simulink model "HVDC_VSC_1CPUcore_dcpl"  (Simulink 8.4)
settings: Solver=ode3  SolverMode=SingleTasking  StartTime=0.0  StopTime=70.0  FixedStep=Ts_Power  RelTol=1e-3  AbsTol=1e-2
PreLoadFcn:
  | Ts_Power=50e-6; Ts_Control=1*Ts_Power; init_cosim_IA; startup_transients_hvdc_vsc;
PostLoadFcn:
  | Ts_Power=50e-6; Ts_Control=1*Ts_Power; init_cosim_IA; startup_transients_hvdc_vsc;
InitFcn:
  | Ts_Power=50e-6; Ts_Control=1*Ts_Power; init_cosim_IA; startup_transients_hvdc_vsc;
undefined symbols (not defined in the file): CLARK, D1, Delta, dPref1_2, dPref1_2_rlimit, gcbh, h, intfDelay, level, lib_mesures, magnitude, ResistanceM, rte_drive_private_lib, rte_tsb3level_hiz_rect_cb, sps_rtmsupport, t_deblock_Pref1, t_deblock_Udref2, t_dPref1_2, t_SwitchITMIdc, t_SwitchITMVdc, Ts_intf, TSB3_hiZR
libraries: powerlib x183, spsVIMeasurementModel x102, powerlib_extras x71, powerlib_meascontrol x50, rteventslib x26, op_dpl_lib x20, rtlab x14, sps_avr x6, artemis x1
(part 3 of 13)

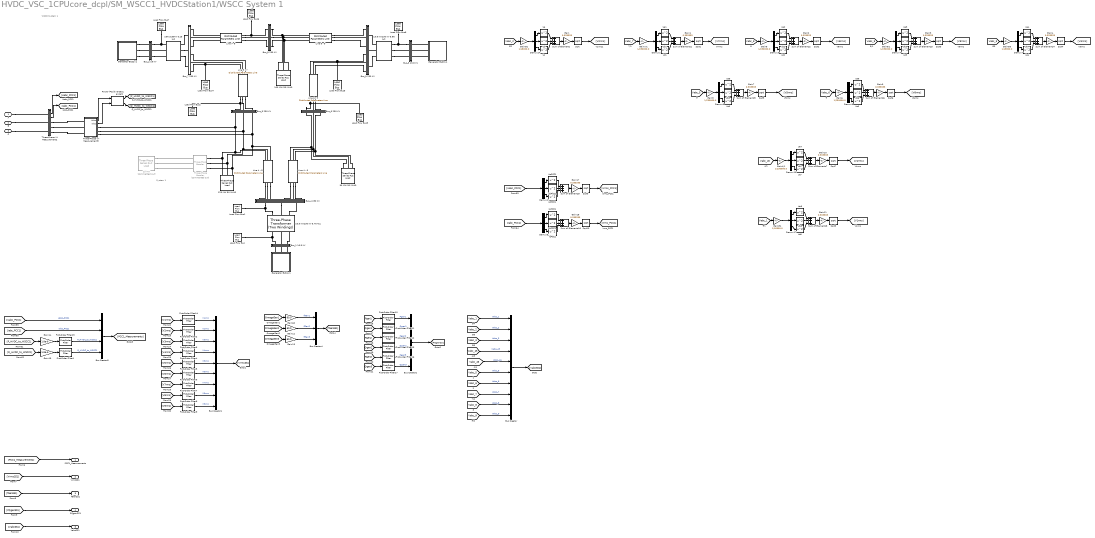
== system HVDC_VSC_1CPUcore_dcpl/SM_WSCC1_HVDCStation1/WSCC System 1 ==
  note: System 1
  note: WSCC System 1
  " Line 4 - 6" : op_dpl_lib/Distributed Parameters Line  SimulationMode=ARTEMIS model  Phases=3  Frequency=60  Resistance=[0.08993 0.224825]  Inductance="[1.41e-3  3.22e-3]"  Capacitance=[7.922e-9 4.74e-9]  Length=100  Measurements=None
  " Line 6 - 9" : op_dpl_lib/Distributed Parameters Line  SimulationMode=ARTEMIS model  Phases=3  Frequency=60  Resistance=[0.20631 0.5157]  Inductance="[2.38e-3  6.09e-3]"  Capacitance=[17.95e-9 10.55e-9]  Length=100  Measurements=None
  100 MW 35 MVAR : powerlib/Elements/Three-Phase Series RLC Load  LConnTagsString=A|B|C  Configuration=Y (grounded)  NominalVoltage=(230000)*1.01601  NominalFrequency=60  ActivePower=100e6  InductivePower=35e6  CapacitivePower=0  Measurements=None  LoadType=constant PQ
  125 MW 50 MVAR : powerlib/Elements/Three-Phase Series RLC Load  LConnTagsString=A|B|C  Configuration=Y (grounded)  NominalVoltage=(230000)*0.996126  NominalFrequency=60  ActivePower=125e6  InductivePower=50e6  CapacitivePower=0  Measurements=None  LoadType=constant PQ
  13.8 KV/230 KV 5.86 %Z : powerlib/Elements/Three-Phase Transformer (Two Windings)  Winding1Connection=Yg  UNITS=pu  NominalPower=[ 128e6 , 60 ]  Winding1=[ 13.8e3 , 1e-6 , 0.0 ]  Winding2Connection=Yg  Winding2=[ 230e3 , 1e-6, 0.075008 ]  SetSaturation=off  Rm=inf  Lm=inf  Saturation=[ 0,0 ; 0.0024,1.2 ; 1.0,1.52 ]  Hysteresis=off  DataFile='hysteresis'  SetInitialFlux=off  InitialFluxes=[ 0.8 , -0.8 , 0.7 ]  Measurements=None  MoreParameters=off  BreakLoop=off  DataType=off  TransfoNumber=1
  "16.5 KV/230 KV 5.76 %Z     " : powerlib/Elements/Three-Phase Transformer (Two Windings)  Winding1Connection=Yg  UNITS=pu  NominalPower=[ 247.5e6 , 60 ]  Winding1=[ 16.5e3 , 1e-6, 0.0 ]  Winding2Connection=Yg  Winding2=[ 230e3 ,1e-6, 0.14256 ]  SetSaturation=off  Rm=inf  Lm=inf  Saturation=[ 0,0 ; 0.0024,1.2 ; 1.0,1.52 ]  Hysteresis=off  DataFile='hysteresis'  SetInitialFlux=off  InitialFluxes=[ 0.8 , -0.8 , 0.7 ]  Measurements=None  MoreParameters=off  BreakLoop=off  DataType=off  TransfoNumber=1
  18KV/230KV 6.25 %Z : powerlib/Elements/Three-Phase Transformer (Two Windings)  Winding1Connection=Yg  UNITS=pu  NominalPower=[ 192e6 , 60 ]  Winding1=[ 18e3 , 1e-6 , 0.0 ]  Winding2Connection=Yg  Winding2=[ 230e3 , 1e-6, 0.12 ]  SetSaturation=off  Rm=inf  Lm=inf  Saturation=[ 0,0 ; 0.0024,1.2 ; 1.0,1.52 ]  Hysteresis=off  DataFile='hysteresis'  SetInitialFlux=off  InitialFluxes=[ 0.8 , -0.8 , 0.7 ]  Measurements=None  MoreParameters=off  BreakLoop=off  DataType=off  TransfoNumber=1
  25 MW : powerlib/Elements/Three-Phase Series RLC Load  Commented=on  LConnTagsString=A|B|C  Configuration=Y (grounded)  NominalVoltage=230000  NominalFrequency=60  ActivePower=25e6  InductivePower=0  CapacitivePower=0  Measurements=None  LoadType=constant PQ
  90 MW 30 MVAR : powerlib/Elements/Three-Phase Series RLC Load  LConnTagsString=A|B|C  Configuration=Y (grounded)  NominalVoltage=(230000)*1.01311  NominalFrequency=60  ActivePower=90e6  InductivePower=30e6  CapacitivePower=0  Measurements=None  LoadType=constant PQ
  Bus Creator : BusCreator  Inputs=10
  Bus Creator1 : BusCreator  Inputs=9
  Bus Creator2 : BusCreator  Inputs=6
  Bus Creator4 : BusCreator  Inputs=3
  Bus Creator5 : BusCreator
  Bus_1 16.5 KV : Subsystem  DialogController=POWERSYS.PowerSysDialog  LoadFcn=sps_rtmsupport('LoadFcn',gcbh);  StartFcn=sps_rtmsupport('StartFcn',gcbh);  StopFcn=sps_rtmsupport('StopFcn',gcbh);  mask(Three-Phase VI Measurement){VoltageMeasurement=phase-to-phase, SetLabelV=on, LabelV=Vabc_1, Vpu=off, VpuLL=off, CurrentMeasurement=yes, SetLabelI=on, LabelI=Iabc_1, Ipu=off, Pbase=100e6, Vbase=16.5e3, OutputType=Complex, PhasorSimulation=off, PSBequivalent=0}
      mask prompts: VoltageMeasurement "Voltage measurement"; SetLabelV "Use a label"; LabelV "Signal label  (use a From block to collect this signal)"; Vpu "Voltages in pu,  based on peak value of nominal phase-to-ground voltage"; VpuLL "Voltages in pu,  based on peak value of nominal phase-to-phase  voltage"; CurrentMeasurement "Current measurement"; SetLabelI "Use a label"; LabelI "Signal label  (use a From block to collect this signal)"; Ipu "Currents in pu"; Pbase "Base power ( VA 3 phase)"; Vbase "Nominal voltage used for pu measurement (Vrms phase-phase) :"; OutputType "Output signals in:"; PhasorSimulation "Phasor simulation (internal use)"; PSBequivalent "Equivalent circuit (internal use)"
      mask help:
      | Ideal three-phase voltage and current measurements.
      |
      | The block can output the voltages and currents in per unit values or in volts and amperes.
      mask init: same as HVDC_VSC_1CPUcore_dcpl/SM_WSCC1_HVDCStation1/B1
      settings: CopyFcn=sps_rtmsupport('CopyFcn',gcbh); powericon('ThreePhaseVIMeasurementCopy',gcb)  DeleteFcn=sps_rtmsupport('DeleteFcn',gcbh);  UndoDeleteFcn=sps_rtmsupport('UndoDeleteFcn',gcbh);  ModelCloseFcn=sps_rtmsupport('ModelCloseFcn',gcbh);  PreSaveFcn="sps_rtmsupport('PreSaveFcn',gcbh);  set_param(gcb,'LinkStatus','restore')"  PostSaveFcn=sps_rtmsupport('PostSaveFcn',gcbh);  NameChangeFcn=sps_rtmsupport('NameChangeFcn',gcbh);  PreCopyFcn=sps_rtmsupport('PreCopyFcn',gcbh);  OpenFcn=sps_rtmsupport('OpenFcn',gcbh, [1 2 4 5 6 7 9 -12 13]);  CloseFcn=sps_rtmsupport('CloseFcn',gcbh);  PreDeleteFcn=sps_rtmsupport('PreDeleteFcn',gcbh);
      mask Help: helpview(psbhelp)
      mask TypeOptions VoltageMeasurement: no | phase-to-ground | phase-to-phase
      mask Callback VoltageMeasurement: powericon('ThreePhaseVIMeasurementCback',gcb,'Vselector');
      mask Callback SetLabelV: powericon('ThreePhaseVIMeasurementCback',gcb,'');
      mask Callback Vpu: powericon('ThreePhaseVIMeasurementCback',gcb,'Vpu');
      mask Callback VpuLL: powericon('ThreePhaseVIMeasurementCback',gcb,'VpuLL');
      mask TypeOptions CurrentMeasurement: no | yes
      mask Callback CurrentMeasurement: powericon('ThreePhaseVIMeasurementCback',gcb,'');
      mask Callback SetLabelI: powericon('ThreePhaseVIMeasurementCback',gcb,'');
      mask Callback LabelI: powericon('ThreePhaseVIMeasurementCback',gcb,'');
      mask Callback Ipu: powericon('ThreePhaseVIMeasurementCback',gcb,'');
      mask TypeOptions OutputType: Complex | Real-Imag | Magnitude-Angle | Magnitude
  Bus_2 18 KV : Subsystem  DialogController=POWERSYS.PowerSysDialog  LoadFcn=sps_rtmsupport('LoadFcn',gcbh);  StartFcn=sps_rtmsupport('StartFcn',gcbh);  StopFcn=sps_rtmsupport('StopFcn',gcbh);  mask(Three-Phase VI Measurement){VoltageMeasurement=phase-to-phase, SetLabelV=on, LabelV=Vabc_2, Vpu=off, VpuLL=off, CurrentMeasurement=yes, SetLabelI=on, LabelI=Iabc_2, Ipu=off, Pbase=100e6, Vbase=18e3, OutputType=Complex, PhasorSimulation=off, PSBequivalent=0}
      mask prompts: VoltageMeasurement "Voltage measurement"; SetLabelV "Use a label"; LabelV "Signal label  (use a From block to collect this signal)"; Vpu "Voltages in pu,  based on peak value of nominal phase-to-ground voltage"; VpuLL "Voltages in pu,  based on peak value of nominal phase-to-phase  voltage"; CurrentMeasurement "Current measurement"; SetLabelI "Use a label"; LabelI "Signal label  (use a From block to collect this signal)"; Ipu "Currents in pu"; Pbase "Base power ( VA 3 phase)"; Vbase "Nominal voltage used for pu measurement (Vrms phase-phase) :"; OutputType "Output signals in:"; PhasorSimulation "Phasor simulation (internal use)"; PSBequivalent "Equivalent circuit (internal use)"
      mask help:
      | Ideal three-phase voltage and current measurements.
      |
      | The block can output the voltages and currents in per unit values or in volts and amperes.
      mask init: same as HVDC_VSC_1CPUcore_dcpl/SM_WSCC1_HVDCStation1/B1
      settings: CopyFcn=sps_rtmsupport('CopyFcn',gcbh); powericon('ThreePhaseVIMeasurementCopy',gcb)  DeleteFcn=sps_rtmsupport('DeleteFcn',gcbh);  UndoDeleteFcn=sps_rtmsupport('UndoDeleteFcn',gcbh);  ModelCloseFcn=sps_rtmsupport('ModelCloseFcn',gcbh);  PreSaveFcn="sps_rtmsupport('PreSaveFcn',gcbh);  set_param(gcb,'LinkStatus','restore')"  PostSaveFcn=sps_rtmsupport('PostSaveFcn',gcbh);  NameChangeFcn=sps_rtmsupport('NameChangeFcn',gcbh);  PreCopyFcn=sps_rtmsupport('PreCopyFcn',gcbh);  OpenFcn=sps_rtmsupport('OpenFcn',gcbh, [1 2 4 5 6 7 9 -12 13]);  CloseFcn=sps_rtmsupport('CloseFcn',gcbh);  PreDeleteFcn=sps_rtmsupport('PreDeleteFcn',gcbh);
      mask Help: helpview(psbhelp)
      mask TypeOptions VoltageMeasurement: no | phase-to-ground | phase-to-phase
      mask Callback VoltageMeasurement: powericon('ThreePhaseVIMeasurementCback',gcb,'Vselector');
      mask Callback SetLabelV: powericon('ThreePhaseVIMeasurementCback',gcb,'');
      mask Callback Vpu: powericon('ThreePhaseVIMeasurementCback',gcb,'Vpu');
      mask Callback VpuLL: powericon('ThreePhaseVIMeasurementCback',gcb,'VpuLL');
      mask TypeOptions CurrentMeasurement: no | yes
      mask Callback CurrentMeasurement: powericon('ThreePhaseVIMeasurementCback',gcb,'');
      mask Callback SetLabelI: powericon('ThreePhaseVIMeasurementCback',gcb,'');
      mask Callback LabelI: powericon('ThreePhaseVIMeasurementCback',gcb,'');
      mask Callback Ipu: powericon('ThreePhaseVIMeasurementCback',gcb,'');
      mask TypeOptions OutputType: Complex | Real-Imag | Magnitude-Angle | Magnitude
  Bus_3 13.8 KV : Subsystem  DialogController=POWERSYS.PowerSysDialog  LoadFcn=sps_rtmsupport('LoadFcn',gcbh);  StartFcn=sps_rtmsupport('StartFcn',gcbh);  StopFcn=sps_rtmsupport('StopFcn',gcbh);  mask(Three-Phase VI Measurement){VoltageMeasurement=phase-to-phase, SetLabelV=on, LabelV=Vabc_3, Vpu=off, VpuLL=off, CurrentMeasurement=yes, SetLabelI=on, LabelI=Iabc_3, Ipu=off, Pbase=100e6, Vbase=13.8e3, OutputType=Complex, PhasorSimulation=off, PSBequivalent=0}
      mask prompts: VoltageMeasurement "Voltage measurement"; SetLabelV "Use a label"; LabelV "Signal label  (use a From block to collect this signal)"; Vpu "Voltages in pu,  based on peak value of nominal phase-to-ground voltage"; VpuLL "Voltages in pu,  based on peak value of nominal phase-to-phase  voltage"; CurrentMeasurement "Current measurement"; SetLabelI "Use a label"; LabelI "Signal label  (use a From block to collect this signal)"; Ipu "Currents in pu"; Pbase "Base power ( VA 3 phase)"; Vbase "Nominal voltage used for pu measurement (Vrms phase-phase) :"; OutputType "Output signals in:"; PhasorSimulation "Phasor simulation (internal use)"; PSBequivalent "Equivalent circuit (internal use)"
      mask help:
      | Ideal three-phase voltage and current measurements.
      |
      | The block can output the voltages and currents in per unit values or in volts and amperes.
      mask init: same as HVDC_VSC_1CPUcore_dcpl/SM_WSCC1_HVDCStation1/B1
      settings: CopyFcn=sps_rtmsupport('CopyFcn',gcbh); powericon('ThreePhaseVIMeasurementCopy',gcb)  DeleteFcn=sps_rtmsupport('DeleteFcn',gcbh);  UndoDeleteFcn=sps_rtmsupport('UndoDeleteFcn',gcbh);  ModelCloseFcn=sps_rtmsupport('ModelCloseFcn',gcbh);  PreSaveFcn="sps_rtmsupport('PreSaveFcn',gcbh);  set_param(gcb,'LinkStatus','restore')"  PostSaveFcn=sps_rtmsupport('PostSaveFcn',gcbh);  NameChangeFcn=sps_rtmsupport('NameChangeFcn',gcbh);  PreCopyFcn=sps_rtmsupport('PreCopyFcn',gcbh);  OpenFcn=sps_rtmsupport('OpenFcn',gcbh, [1 2 4 5 6 7 9 -12 13]);  CloseFcn=sps_rtmsupport('CloseFcn',gcbh);  PreDeleteFcn=sps_rtmsupport('PreDeleteFcn',gcbh);
      mask Help: helpview(psbhelp)
      mask TypeOptions VoltageMeasurement: no | phase-to-ground | phase-to-phase
      mask Callback VoltageMeasurement: powericon('ThreePhaseVIMeasurementCback',gcb,'Vselector');
      mask Callback SetLabelV: powericon('ThreePhaseVIMeasurementCback',gcb,'');
      mask Callback Vpu: powericon('ThreePhaseVIMeasurementCback',gcb,'Vpu');
      mask Callback VpuLL: powericon('ThreePhaseVIMeasurementCback',gcb,'VpuLL');
      mask TypeOptions CurrentMeasurement: no | yes
      mask Callback CurrentMeasurement: powericon('ThreePhaseVIMeasurementCback',gcb,'');
      mask Callback SetLabelI: powericon('ThreePhaseVIMeasurementCback',gcb,'');
      mask Callback LabelI: powericon('ThreePhaseVIMeasurementCback',gcb,'');
      mask Callback Ipu: powericon('ThreePhaseVIMeasurementCback',gcb,'');
      mask TypeOptions OutputType: Complex | Real-Imag | Magnitude-Angle | Magnitude
  Bus_4 230 KV : Subsystem
  Bus_5 230 KV : Subsystem  DialogController=POWERSYS.PowerSysDialog  LoadFcn=sps_rtmsupport('LoadFcn',gcbh);  StartFcn=sps_rtmsupport('StartFcn',gcbh);  StopFcn=sps_rtmsupport('StopFcn',gcbh);  mask(Three-Phase VI Measurement){VoltageMeasurement=phase-to-phase, SetLabelV=on, LabelV=Vabc_5, Vpu=off, VpuLL=off, CurrentMeasurement=yes, SetLabelI=on, LabelI=Iabc_5, Ipu=off, Pbase=100e6, Vbase=230e3, OutputType=Complex, PhasorSimulation=off, PSBequivalent=0}
      mask prompts: VoltageMeasurement "Voltage measurement"; SetLabelV "Use a label"; LabelV "Signal label  (use a From block to collect this signal)"; Vpu "Voltages in pu,  based on peak value of nominal phase-to-ground voltage"; VpuLL "Voltages in pu,  based on peak value of nominal phase-to-phase  voltage"; CurrentMeasurement "Current measurement"; SetLabelI "Use a label"; LabelI "Signal label  (use a From block to collect this signal)"; Ipu "Currents in pu"; Pbase "Base power ( VA 3 phase)"; Vbase "Nominal voltage used for pu measurement (Vrms phase-phase) :"; OutputType "Output signals in:"; PhasorSimulation "Phasor simulation (internal use)"; PSBequivalent "Equivalent circuit (internal use)"
      mask help:
      | Ideal three-phase voltage and current measurements.
      |
      | The block can output the voltages and currents in per unit values or in volts and amperes.
      mask init: same as HVDC_VSC_1CPUcore_dcpl/SM_WSCC1_HVDCStation1/B1
      settings: CopyFcn=sps_rtmsupport('CopyFcn',gcbh); powericon('ThreePhaseVIMeasurementCopy',gcb)  DeleteFcn=sps_rtmsupport('DeleteFcn',gcbh);  UndoDeleteFcn=sps_rtmsupport('UndoDeleteFcn',gcbh);  ModelCloseFcn=sps_rtmsupport('ModelCloseFcn',gcbh);  PreSaveFcn="sps_rtmsupport('PreSaveFcn',gcbh);  set_param(gcb,'LinkStatus','restore')"  PostSaveFcn=sps_rtmsupport('PostSaveFcn',gcbh);  NameChangeFcn=sps_rtmsupport('NameChangeFcn',gcbh);  PreCopyFcn=sps_rtmsupport('PreCopyFcn',gcbh);  OpenFcn=sps_rtmsupport('OpenFcn',gcbh, [1 2 4 5 6 7 9 -12 13]);  CloseFcn=sps_rtmsupport('CloseFcn',gcbh);  PreDeleteFcn=sps_rtmsupport('PreDeleteFcn',gcbh);
      mask Help: helpview(psbhelp)
      mask TypeOptions VoltageMeasurement: no | phase-to-ground | phase-to-phase
      mask Callback VoltageMeasurement: powericon('ThreePhaseVIMeasurementCback',gcb,'Vselector');
      mask Callback SetLabelV: powericon('ThreePhaseVIMeasurementCback',gcb,'');
      mask Callback Vpu: powericon('ThreePhaseVIMeasurementCback',gcb,'Vpu');
      mask Callback VpuLL: powericon('ThreePhaseVIMeasurementCback',gcb,'VpuLL');
      mask TypeOptions CurrentMeasurement: no | yes
      mask Callback CurrentMeasurement: powericon('ThreePhaseVIMeasurementCback',gcb,'');
      mask Callback SetLabelI: powericon('ThreePhaseVIMeasurementCback',gcb,'');
      mask Callback LabelI: powericon('ThreePhaseVIMeasurementCback',gcb,'');
      mask Callback Ipu: powericon('ThreePhaseVIMeasurementCback',gcb,'');
      mask TypeOptions OutputType: Complex | Real-Imag | Magnitude-Angle | Magnitude
  Bus_6 230 KV : Subsystem  DialogController=POWERSYS.PowerSysDialog  LoadFcn=sps_rtmsupport('LoadFcn',gcbh);  StartFcn=sps_rtmsupport('StartFcn',gcbh);  StopFcn=sps_rtmsupport('StopFcn',gcbh);  mask(Three-Phase VI Measurement){VoltageMeasurement=phase-to-phase, SetLabelV=on, LabelV=Vabc_6, Vpu=off, VpuLL=off, CurrentMeasurement=yes, SetLabelI=on, LabelI=Iabc_6, Ipu=off, Pbase=100e6, Vbase=230e3, OutputType=Complex, PhasorSimulation=off, PSBequivalent=0}
      mask prompts: VoltageMeasurement "Voltage measurement"; SetLabelV "Use a label"; LabelV "Signal label  (use a From block to collect this signal)"; Vpu "Voltages in pu,  based on peak value of nominal phase-to-ground voltage"; VpuLL "Voltages in pu,  based on peak value of nominal phase-to-phase  voltage"; CurrentMeasurement "Current measurement"; SetLabelI "Use a label"; LabelI "Signal label  (use a From block to collect this signal)"; Ipu "Currents in pu"; Pbase "Base power ( VA 3 phase)"; Vbase "Nominal voltage used for pu measurement (Vrms phase-phase) :"; OutputType "Output signals in:"; PhasorSimulation "Phasor simulation (internal use)"; PSBequivalent "Equivalent circuit (internal use)"
      mask help:
      | Ideal three-phase voltage and current measurements.
      |
      | The block can output the voltages and currents in per unit values or in volts and amperes.
      mask init: same as HVDC_VSC_1CPUcore_dcpl/SM_WSCC1_HVDCStation1/B1
      settings: CopyFcn=sps_rtmsupport('CopyFcn',gcbh); powericon('ThreePhaseVIMeasurementCopy',gcb)  DeleteFcn=sps_rtmsupport('DeleteFcn',gcbh);  UndoDeleteFcn=sps_rtmsupport('UndoDeleteFcn',gcbh);  ModelCloseFcn=sps_rtmsupport('ModelCloseFcn',gcbh);  PreSaveFcn="sps_rtmsupport('PreSaveFcn',gcbh);  set_param(gcb,'LinkStatus','restore')"  PostSaveFcn=sps_rtmsupport('PostSaveFcn',gcbh);  NameChangeFcn=sps_rtmsupport('NameChangeFcn',gcbh);  PreCopyFcn=sps_rtmsupport('PreCopyFcn',gcbh);  OpenFcn=sps_rtmsupport('OpenFcn',gcbh, [1 2 4 5 6 7 9 -12 13]);  CloseFcn=sps_rtmsupport('CloseFcn',gcbh);  PreDeleteFcn=sps_rtmsupport('PreDeleteFcn',gcbh);
      mask Help: helpview(psbhelp)
      mask TypeOptions VoltageMeasurement: no | phase-to-ground | phase-to-phase
      mask Callback VoltageMeasurement: powericon('ThreePhaseVIMeasurementCback',gcb,'Vselector');
      mask Callback SetLabelV: powericon('ThreePhaseVIMeasurementCback',gcb,'');
      mask Callback Vpu: powericon('ThreePhaseVIMeasurementCback',gcb,'Vpu');
      mask Callback VpuLL: powericon('ThreePhaseVIMeasurementCback',gcb,'VpuLL');
      mask TypeOptions CurrentMeasurement: no | yes
      mask Callback CurrentMeasurement: powericon('ThreePhaseVIMeasurementCback',gcb,'');
      mask Callback SetLabelI: powericon('ThreePhaseVIMeasurementCback',gcb,'');
      mask Callback LabelI: powericon('ThreePhaseVIMeasurementCback',gcb,'');
      mask Callback Ipu: powericon('ThreePhaseVIMeasurementCback',gcb,'');
      mask TypeOptions OutputType: Complex | Real-Imag | Magnitude-Angle | Magnitude
  Bus_7 230 KV : Subsystem
  Bus_8 230 KV : Subsystem  DialogController=POWERSYS.PowerSysDialog  LoadFcn=sps_rtmsupport('LoadFcn',gcbh);  StartFcn=sps_rtmsupport('StartFcn',gcbh);  StopFcn=sps_rtmsupport('StopFcn',gcbh);  mask(Three-Phase VI Measurement){VoltageMeasurement=phase-to-phase, SetLabelV=on, LabelV=Vabc_8, Vpu=off, VpuLL=off, CurrentMeasurement=yes, SetLabelI=on, LabelI=Iabc_8, Ipu=off, Pbase=100e6, Vbase=230e3, OutputType=Complex, PhasorSimulation=off, PSBequivalent=0}
      mask prompts: VoltageMeasurement "Voltage measurement"; SetLabelV "Use a label"; LabelV "Signal label  (use a From block to collect this signal)"; Vpu "Voltages in pu,  based on peak value of nominal phase-to-ground voltage"; VpuLL "Voltages in pu,  based on peak value of nominal phase-to-phase  voltage"; CurrentMeasurement "Current measurement"; SetLabelI "Use a label"; LabelI "Signal label  (use a From block to collect this signal)"; Ipu "Currents in pu"; Pbase "Base power ( VA 3 phase)"; Vbase "Nominal voltage used for pu measurement (Vrms phase-phase) :"; OutputType "Output signals in:"; PhasorSimulation "Phasor simulation (internal use)"; PSBequivalent "Equivalent circuit (internal use)"
      mask help:
      | Ideal three-phase voltage and current measurements.
      |
      | The block can output the voltages and currents in per unit values or in volts and amperes.
      mask init: same as HVDC_VSC_1CPUcore_dcpl/SM_WSCC1_HVDCStation1/B1
      settings: CopyFcn=sps_rtmsupport('CopyFcn',gcbh); powericon('ThreePhaseVIMeasurementCopy',gcb)  DeleteFcn=sps_rtmsupport('DeleteFcn',gcbh);  UndoDeleteFcn=sps_rtmsupport('UndoDeleteFcn',gcbh);  ModelCloseFcn=sps_rtmsupport('ModelCloseFcn',gcbh);  PreSaveFcn="sps_rtmsupport('PreSaveFcn',gcbh);  set_param(gcb,'LinkStatus','restore')"  PostSaveFcn=sps_rtmsupport('PostSaveFcn',gcbh);  NameChangeFcn=sps_rtmsupport('NameChangeFcn',gcbh);  PreCopyFcn=sps_rtmsupport('PreCopyFcn',gcbh);  OpenFcn=sps_rtmsupport('OpenFcn',gcbh, [1 2 4 5 6 7 9 -12 13]);  CloseFcn=sps_rtmsupport('CloseFcn',gcbh);  PreDeleteFcn=sps_rtmsupport('PreDeleteFcn',gcbh);
      mask Help: helpview(psbhelp)
      mask TypeOptions VoltageMeasurement: no | phase-to-ground | phase-to-phase
      mask Callback VoltageMeasurement: powericon('ThreePhaseVIMeasurementCback',gcb,'Vselector');
      mask Callback SetLabelV: powericon('ThreePhaseVIMeasurementCback',gcb,'');
      mask Callback Vpu: powericon('ThreePhaseVIMeasurementCback',gcb,'Vpu');
      mask Callback VpuLL: powericon('ThreePhaseVIMeasurementCback',gcb,'VpuLL');
      mask TypeOptions CurrentMeasurement: no | yes
      mask Callback CurrentMeasurement: powericon('ThreePhaseVIMeasurementCback',gcb,'');
      mask Callback SetLabelI: powericon('ThreePhaseVIMeasurementCback',gcb,'');
      mask Callback LabelI: powericon('ThreePhaseVIMeasurementCback',gcb,'');
      mask Callback Ipu: powericon('ThreePhaseVIMeasurementCback',gcb,'');
      mask TypeOptions OutputType: Complex | Real-Imag | Magnitude-Angle | Magnitude
  Bus_9 230 KV : Subsystem
  Demux{1..7,9..10,17,24} (11 alike) : Demux  Outputs=3
  First-Order Filter{1..17} (17 alike) : powerlib_meascontrol/Filters/First-Order Filter  FilterType=Lowpass  Tc=0.05  Ts=Ts_Power  Initialize=on  Vac_Init=[0, 0, 0]  Vdc_Init=0  PlotResponse=off  FreqRange="[0,  200,  1]"
  Gain{,1..4,7,9..11,17..18} (11 alike) : Gain  Gain=0.333333
  Gain12 : Gain  Gain=60.0
  Gain13 : Gain  Gain=60.0
  Gain14 : Gain  Gain=1.0e-6
  Gain15 : Gain  Gain=1.0e-6
  Gain4/1 : Gain  Gain=1/230000.0
  Gain5 : Gain  Gain=1/230000.0
  Gain6 : Gain  Gain=1/230000.0
  Gain60 : Gain  Gain=60.0
  Gain7/1 : Gain  Gain=1/230000.0
  Gain8 : Gain  Gain=1/230000.0
  Gain9/1 : Gain  Gain=1/230000.0
  GainG1 : Gain  Gain=1/16500.0
  GainG2 : Gain  Gain=1/18000.0
  GainG3 : Gain  Gain=1/13800.0
  Generator BUS1x1 : Subsystem
  Generator BUS2x1 : Subsystem
  Generator BUS3x1 : Subsystem
  IaPCC1 : Math  Operator=square  SaturateOnIntegerOverflow=on
  IbPCC1 : Math  Operator=square  SaturateOnIntegerOverflow=on
  IcPCC1 : Math  Operator=square  SaturateOnIntegerOverflow=on
  "Line 4 - 5 " : op_dpl_lib/Distributed Parameters Line  SimulationMode=ARTEMIS model  Phases=3  Frequency=60  Resistance=[0.0529 0.13225]  Inductance="[1.2599e-3  2.38e-3]"  Capacitance=[8.82e-9 5.188e-9]  Length=100  Measurements=None
  "Line 5 - 7 " : op_dpl_lib/Distributed Parameters Line  SimulationMode=ARTEMIS model  Phases=3  Frequency=60  Resistance=[0.16928 0.4232]  Inductance="[2.259e-3  5.64e-3]"  Capacitance=[15.34e-9 9.025e-9]  Length=100  Measurements=None
  Line 7- 8 : op_dpl_lib/Distributed Parameters Line  SimulationMode=ARTEMIS model  Phases=3  Frequency=60  Resistance=[0.044965 0.8768175]  Inductance=[1.488e-3 1.488e-3]  Capacitance=[7.471e-9 7.471e-9]  Length=100  Measurements=None
  Line 8 - 9 : op_dpl_lib/Distributed Parameters Line  SimulationMode=ARTEMIS model  Phases=3  Frequency=60  Resistance=[0.062951 0.15737]  Inductance="[1.414e-3  3.53e-3]"  Capacitance=[10.47e-9 6.15e-9]  Length=100  Measurements=None
  Load Flow Bus : powerlib/Measurements/Load Flow Bus  LConnTagsString=a  ID=BUS_1  Vbase=16.5e3  Vref=1.04  Vangle=0  VLF=1.04  angleLF=0
      settings: AttributesFormatString=%<ID>\n%<Vbase>V\n%<VLF>pu\n%<angleLF>deg.
  Load Flow Bus1 : powerlib/Measurements/Load Flow Bus  LConnTagsString=a  ID=BUS_4  Vbase=230e3  Vref=1  Vangle=0  VLF=1.026  angleLF=-2.214
      settings: AttributesFormatString=%<ID>\n%<Vbase>V\n%<VLF>pu\n%<angleLF>deg.
  Load Flow Bus2 : powerlib/Measurements/Load Flow Bus  LConnTagsString=a  ID=BUS_5  Vbase=230e3  Vref=1  Vangle=0  VLF=0.9961  angleLF=-3.98
      settings: AttributesFormatString=%<ID>\n%<Vbase>V\n%<VLF>pu\n%<angleLF>deg.
  Load Flow Bus3 : powerlib/Measurements/Load Flow Bus  LConnTagsString=a  ID=BUS_6  Vbase=230e3  Vref=1  Vangle=0  VLF=1.013  angleLF=-3.678
      settings: AttributesFormatString=%<ID>\n%<Vbase>V\n%<VLF>pu\n%<angleLF>deg.
  Load Flow Bus4 : powerlib/Measurements/Load Flow Bus  LConnTagsString=a  ID=BUS_7  Vbase=230e3  Vref=1  Vangle=0  VLF=1.026  angleLF=3.662
      settings: AttributesFormatString=%<ID>\n%<Vbase>V\n%<VLF>pu\n%<angleLF>deg.
  Load Flow Bus5 : powerlib/Measurements/Load Flow Bus  LConnTagsString=a  ID=BUS_9  Vbase=230e3  Vref=1  Vangle=0  VLF=1.032  angleLF=1.909
      settings: AttributesFormatString=%<ID>\n%<Vbase>V\n%<VLF>pu\n%<angleLF>deg.
  Load Flow Bus6 : powerlib/Measurements/Load Flow Bus  LConnTagsString=a  ID=BUS_8  Vbase=230e3  Vref=1  Vangle=0  VLF=1.016  angleLF=0.6755
      settings: AttributesFormatString=%<ID>\n%<Vbase>V\n%<VLF>pu\n%<angleLF>deg.
  Load Flow Bus7 : powerlib/Measurements/Load Flow Bus  LConnTagsString=a  ID=BUS_2  Vbase=18e3  Vref=1.025  Vangle=0  VLF=1.025  angleLF=9.222
      settings: AttributesFormatString=%<ID>\n%<Vbase>V\n%<VLF>pu\n%<angleLF>deg.
  Load Flow Bus8 : powerlib/Measurements/Load Flow Bus  LConnTagsString=a  ID=BUS_3  Vbase=13.8e3  Vref=1.025  Vangle=4.7  VLF=1.025  angleLF=4.606
      settings: AttributesFormatString=%<ID>\n%<Vbase>V\n%<VLF>pu\n%<angleLF>deg.
  Power (Positive-Sequence)2 : powerlib_meascontrol/Measurements/Power (Positive-Sequence)  Freq=60  Vinit=[0, 0]  Iinit=[0, 0]  Ts=0
  Sqrt{,1..10} (11 alike) : Sqrt  SaturateOnIntegerOverflow=on
  Sum of Elements{,1..10} (11 alike) : Sum  Inputs=+|+|+
  Three-Phase V-I Measurement2 : Subsystem  DialogController=POWERSYS.PowerSysDialog  LoadFcn=sps_rtmsupport('LoadFcn',gcbh);  StartFcn=sps_rtmsupport('StartFcn',gcbh);  StopFcn=sps_rtmsupport('StopFcn',gcbh);  mask(Three-Phase VI Measurement){VoltageMeasurement=phase-to-ground, SetLabelV=off, LabelV=Vabc, Vpu=off, VpuLL=off, CurrentMeasurement=yes, SetLabelI=off, LabelI=Iabc, Ipu=off, Pbase=100e6, Vbase=500e3, OutputType=Complex, PhasorSimulation=off, PSBequivalent=0}
      mask prompts: VoltageMeasurement "Voltage measurement"; SetLabelV "Use a label"; LabelV "Signal label  (use a From block to collect this signal)"; Vpu "Voltages in pu,  based on peak value of nominal phase-to-ground voltage"; VpuLL "Voltages in pu,  based on peak value of nominal phase-to-phase  voltage"; CurrentMeasurement "Current measurement"; SetLabelI "Use a label"; LabelI "Signal label  (use a From block to collect this signal)"; Ipu "Currents in pu"; Pbase "Base power ( VA 3 phase)"; Vbase "Nominal voltage used for pu measurement (Vrms phase-phase) :"; OutputType "Output signals in:"; PhasorSimulation "Phasor simulation (internal use)"; PSBequivalent "Equivalent circuit (internal use)"
      mask help:
      | Ideal three-phase voltage and current measurements.
      |
      | The block can output the voltages and currents in per unit values or in volts and amperes.
      mask init: same as HVDC_VSC_1CPUcore_dcpl/SM_WSCC1_HVDCStation1/B1
      settings: CopyFcn=sps_rtmsupport('CopyFcn',gcbh); powericon('ThreePhaseVIMeasurementCopy',gcb)  DeleteFcn=sps_rtmsupport('DeleteFcn',gcbh);  UndoDeleteFcn=sps_rtmsupport('UndoDeleteFcn',gcbh);  ModelCloseFcn=sps_rtmsupport('ModelCloseFcn',gcbh);  PreSaveFcn="sps_rtmsupport('PreSaveFcn',gcbh);  set_param(gcb,'LinkStatus','restore')"  PostSaveFcn=sps_rtmsupport('PostSaveFcn',gcbh);  NameChangeFcn=sps_rtmsupport('NameChangeFcn',gcbh);  PreCopyFcn=sps_rtmsupport('PreCopyFcn',gcbh);  OpenFcn=sps_rtmsupport('OpenFcn',gcbh, [1 2 4 5 6 7 9 -12 13]);  CloseFcn=sps_rtmsupport('CloseFcn',gcbh);  PreDeleteFcn=sps_rtmsupport('PreDeleteFcn',gcbh);
      mask Help: helpview(psbhelp)
      mask TypeOptions VoltageMeasurement: no | phase-to-ground | phase-to-phase
      mask Callback VoltageMeasurement: powericon('ThreePhaseVIMeasurementCback',gcb,'Vselector');
      mask Callback SetLabelV: powericon('ThreePhaseVIMeasurementCback',gcb,'');
      mask Callback Vpu: powericon('ThreePhaseVIMeasurementCback',gcb,'Vpu');
      mask Callback VpuLL: powericon('ThreePhaseVIMeasurementCback',gcb,'VpuLL');
      mask TypeOptions CurrentMeasurement: no | yes
      mask Callback CurrentMeasurement: powericon('ThreePhaseVIMeasurementCback',gcb,'');
      mask Callback SetLabelI: powericon('ThreePhaseVIMeasurementCback',gcb,'');
      mask Callback LabelI: powericon('ThreePhaseVIMeasurementCback',gcb,'');
      mask Callback Ipu: powericon('ThreePhaseVIMeasurementCback',gcb,'');
      mask TypeOptions OutputType: Complex | Real-Imag | Magnitude-Angle | Magnitude
  Three-Phase V-I Measurement3 : Subsystem  DialogController=POWERSYS.PowerSysDialog  LoadFcn=sps_rtmsupport('LoadFcn',gcbh);  StartFcn=sps_rtmsupport('StartFcn',gcbh);  StopFcn=sps_rtmsupport('StopFcn',gcbh);  mask(Three-Phase VI Measurement){VoltageMeasurement=phase-to-ground, SetLabelV=off, LabelV=Vabc, Vpu=off, VpuLL=off, CurrentMeasurement=yes, SetLabelI=off, LabelI=Iabc, Ipu=off, Pbase=100e6, Vbase=500e3, OutputType=Complex, PhasorSimulation=off, PSBequivalent=0}
      mask prompts: VoltageMeasurement "Voltage measurement"; SetLabelV "Use a label"; LabelV "Signal label  (use a From block to collect this signal)"; Vpu "Voltages in pu,  based on peak value of nominal phase-to-ground voltage"; VpuLL "Voltages in pu,  based on peak value of nominal phase-to-phase  voltage"; CurrentMeasurement "Current measurement"; SetLabelI "Use a label"; LabelI "Signal label  (use a From block to collect this signal)"; Ipu "Currents in pu"; Pbase "Base power ( VA 3 phase)"; Vbase "Nominal voltage used for pu measurement (Vrms phase-phase) :"; OutputType "Output signals in:"; PhasorSimulation "Phasor simulation (internal use)"; PSBequivalent "Equivalent circuit (internal use)"
      mask help:
      | Ideal three-phase voltage and current measurements.
      |
      | The block can output the voltages and currents in per unit values or in volts and amperes.
      mask init: same as HVDC_VSC_1CPUcore_dcpl/SM_WSCC1_HVDCStation1/B1
      settings: CopyFcn=sps_rtmsupport('CopyFcn',gcbh); powericon('ThreePhaseVIMeasurementCopy',gcb)  DeleteFcn=sps_rtmsupport('DeleteFcn',gcbh);  UndoDeleteFcn=sps_rtmsupport('UndoDeleteFcn',gcbh);  ModelCloseFcn=sps_rtmsupport('ModelCloseFcn',gcbh);  PreSaveFcn="sps_rtmsupport('PreSaveFcn',gcbh);  set_param(gcb,'LinkStatus','restore')"  PostSaveFcn=sps_rtmsupport('PostSaveFcn',gcbh);  NameChangeFcn=sps_rtmsupport('NameChangeFcn',gcbh);  PreCopyFcn=sps_rtmsupport('PreCopyFcn',gcbh);  OpenFcn=sps_rtmsupport('OpenFcn',gcbh, [1 2 4 5 6 7 9 -12 13]);  CloseFcn=sps_rtmsupport('CloseFcn',gcbh);  PreDeleteFcn=sps_rtmsupport('PreDeleteFcn',gcbh);
      mask Help: helpview(psbhelp)
      mask TypeOptions VoltageMeasurement: no | phase-to-ground | phase-to-phase
      mask Callback VoltageMeasurement: powericon('ThreePhaseVIMeasurementCback',gcb,'Vselector');
      mask Callback SetLabelV: powericon('ThreePhaseVIMeasurementCback',gcb,'');
      mask Callback Vpu: powericon('ThreePhaseVIMeasurementCback',gcb,'Vpu');
      mask Callback VpuLL: powericon('ThreePhaseVIMeasurementCback',gcb,'VpuLL');
      mask TypeOptions CurrentMeasurement: no | yes
      mask Callback CurrentMeasurement: powericon('ThreePhaseVIMeasurementCback',gcb,'');
      mask Callback SetLabelI: powericon('ThreePhaseVIMeasurementCback',gcb,'');
      mask Callback LabelI: powericon('ThreePhaseVIMeasurementCback',gcb,'');
      mask Callback Ipu: powericon('ThreePhaseVIMeasurementCback',gcb,'');
      mask TypeOptions OutputType: Complex | Real-Imag | Magnitude-Angle | Magnitude
  Three-Phase Breaker : powerlib/Elements/Three-Phase Breaker  Commented=on  InitialState=open  SwitchA=on  SwitchB=on  SwitchC=on  SwitchTimes=[ 50.0 ]  External=off  BreakerResistance=0.01  SnubberResistance=1e6  SnubberCapacitance=inf  Measurements=None
  Ua{,1..8} (9 alike) : Math  Operator=square  SaturateOnIntegerOverflow=on
  UaPCC1 : Math  Operator=square  SaturateOnIntegerOverflow=on
  Ub{,1..8} (9 alike) : Math  Operator=square  SaturateOnIntegerOverflow=on
  UbPCC1 : Math  Operator=square  SaturateOnIntegerOverflow=on
  Uc{,1..8} (9 alike) : Math  Operator=square  SaturateOnIntegerOverflow=on
  UcPCC1 : Math  Operator=square  SaturateOnIntegerOverflow=on
  A : PMIOPort  Port=1  Side=Left
  B : PMIOPort  Port=2  Side=Left
  C : PMIOPort  Port=3  Side=Left
  PCC1_Measurements : Outport
  VrmsSS1 : Outport  Port=2
  fGenSS1 : Outport  Port=3
  PQgenSS1 : Outport  Port=4
  VabcSS1 : Outport  Port=5
  wires:
  Bus Creator/1 -> [VabcSS1]
  [Vabc_5] -> Gain5/1
  Bus Creator2/1 -> [PQgenSS1]
  [Vabc_3] -> GainG3/1
  [Vabc_9] -> Gain9/1/1
  Gain/1 -> Sqrt/1
  Gain1/1 -> Sqrt1/1
  Gain4/1 -> Sqrt4/1
  Ua4/1 -> Sum of Elements4/1
  Demux3/1 -> Ua2/1
  Gain5/1 -> Demux6/1
  [Vabc_8] -> Gain8/1
  Ub3/1 -> Sum of Elements3/2
  [Vabc_7] -> Gain7/1/1
  Sqrt7/1 -> [V4rms]
  Ub5/1 -> Sum of Elements5/2
  Sum of Elements1/1 -> Gain1/1
  Ua3/1 -> Sum of Elements3/1
  Uc3/1 -> Sum of Elements3/3
  Demux7/3 -> Uc4/1
  [Vabc_2] -> GainG2/1
  Demux2/1 -> Ua1/1
  Sqrt1/1 -> [V7rms]
  Ub1/1 -> Sum of Elements1/2
  Sqrt/1 -> [V2rms]
  Demux24/2 -> Ub/1
  Demux24/1 -> Ua/1
  [Vabc_6] -> Gain6/1
  Ua/1 -> Sum of Elements/1
  Sum of Elements/1 -> Gain/1
  Demux24/3 -> Uc/1
  Sum of Elements4/1 -> Gain4/1
  Sqrt2/1 -> [V8rms]
  Uc/1 -> Sum of Elements/3
  Demux2/2 -> Ub1/1
  Demux6/1 -> Ua5/1
  Gain2/1 -> Sqrt2/1
  [Vabc_1] -> GainG1/1
  Ub/1 -> Sum of Elements/2
  Gain7/1/1 -> Demux2/1
  Uc1/1 -> Sum of Elements1/3
  [Vabc_45] -> Gain4/1/1
  Demux2/3 -> Uc1/1
  Demux3/3 -> Uc2/1
  Ua1/1 -> Sum of Elements1/1
  GainG2/1 -> Demux24/1
  Demux10/2 -> Ub7/1
  Demux7/1 -> Ua4/1
  GainG3/1 -> Demux7/1
  Demux4/3 -> Uc3/1
  Demux6/3 -> Uc5/1
  Sum of Elements5/1 -> Gain7/1
  Uc5/1 -> Sum of Elements5/3
  Sqrt3/1 -> [V9rms]
  Gain7/1 -> Sqrt5/1
  Ua8/1 -> Sum of Elements8/1
  Gain4/1/1 -> Demux10/1
  Demux4/2 -> Ub3/1
  Uc2/1 -> Sum of Elements2/3
  Sum of Elements2/1 -> Gain2/1
  Demux6/2 -> Ub5/1
  Ub4/1 -> Sum of Elements4/2
  Demux3/2 -> Ub2/1
  Gain9/1/1 -> Demux4/1
  Ub2/1 -> Sum of Elements2/2
  Demux17/1 -> Ua8/1
  Sqrt8/1 -> [V1rms]
  Sqrt4/1 -> [V3rms]
  Ua6/1 -> Sum of Elements6/1
  Ua5/1 -> Sum of Elements5/1
  Sum of Elements3/1 -> Gain3/1
  Gain3/1 -> Sqrt3/1
  Gain6/1 -> Demux9/1
  Gain8/1 -> Demux3/1
  Demux7/2 -> Ub4/1
  Uc4/1 -> Sum of Elements4/3
  Demux4/1 -> Ua3/1
  Demux9/2 -> Ub6/1
  Uc8/1 -> Sum of Elements8/3
  Demux9/3 -> Uc6/1
  Ua7/1 -> Sum of Elements7/1
  Gain11/1 -> Sqrt8/1
  Gain10/1 -> Sqrt7/1
  Sum of Elements7/1 -> Gain10/1
  [V2rms] -> First-Order Filter2/1
  [V4rms] -> First-Order Filter4/1
  Demux10/3 -> Uc7/1
  [Vabc_3] -> Bus Creator/3  "Vabc_3"
  [Qgen1] -> First-Order Filter11/1
  Ub8/1 -> Sum of Elements8/2
  Ub6/1 -> Sum of Elements6/2
  Uc6/1 -> Sum of Elements6/3
  Demux9/1 -> Ua6/1
  Ua2/1 -> Sum of Elements2/1
  [Vabc_9] -> Bus Creator/10  "Vabc_9"
  [V9rms] -> First-Order Filter9/1
  Bus Creator1/1 -> [VrmsSS1]
  [V6rms] -> First-Order Filter6/1
  Uc7/1 -> Sum of Elements7/3
  [V1rms] -> First-Order Filter14/1
  Demux10/1 -> Ua7/1
  [V7rms] -> First-Order Filter7/1
  Sum of Elements6/1 -> Gain9/1
  GainG1/1 -> Demux17/1
  Ub7/1 -> Sum of Elements7/2
  Sqrt6/1 -> [V6rms]
  Demux17/2 -> Ub8/1
  Sum of Elements8/1 -> Gain11/1
  Demux17/3 -> Uc8/1
  Gain9/1 -> Sqrt6/1
  [V3rms] -> First-Order Filter3/1
  Three-Phase V-I Measurement2/2(Iabc) -> [Iabc_PCC1]
  Three-Phase V-I Measurement3/1(Vabc) -> Power (Positive-Sequence)2/1
  [Vabc_8] -> Bus Creator/9  "Vabc_8"
  [OmegaGen2] -> Gain12/1
  [OmegaGen3] -> Gain13/1
  [Vabc_45] -> Bus Creator/4  "Vabc_45"
  [V5rms] -> First-Order Filter5/1
  Power (Positive-Sequence)2/2 -> [Q_HVDC_to_WSCC1]
  [Pgen2] -> First-Order Filter12/1
  Gain13/1 -> Bus Creator4/3  "fGen3"
  [Pgen1] -> First-Order Filter10/1
  Three-Phase V-I Measurement3/2(Iabc) -> Power (Positive-Sequence)2/2
  Gain12/1 -> Bus Creator4/2  "fGen2"
  [V8rms] -> First-Order Filter8/1
  Sqrt5/1 -> [V5rms]
  [Vabc_6] -> Bus Creator/7  "Vabc_6"
  [OmegaGen1] -> Gain60/1
  Gain60/1 -> Bus Creator4/1  "fGen1"
  Power (Positive-Sequence)2/1 -> [P_HVDC_to_WSCC1]
  Bus Creator4/1 -> [fGenSS1]
  [Vabc_1] -> Bus Creator/1  "Vabc_1"
  [Vabc_2] -> Bus Creator/2  "Vabc_2"
  [Vabc_5] -> Bus Creator/6  "Vabc_5"
  [Vabc_7] -> Bus Creator/8  "Vabc_7"
  Three-Phase V-I Measurement2/1(Vabc) -> [Uabc_PCC1]
  [Vabc_46] -> Bus Creator/5  "Vabc_46"
  [Qgen3] -> First-Order Filter17/1
  [Pgen3] -> First-Order Filter16/1
  [Qgen2] -> First-Order Filter13/1
  Bus Creator5/1 -> [PCC1_Measurements]
  Gain17/1 -> Sqrt9/1
  UcPCC1/1 -> Sum of Elements9/3
  IbPCC1/1 -> Sum of Elements10/2
  Demux1/2 -> UbPCC1/1
  IaPCC1/1 -> Sum of Elements10/1
  Sqrt9/1 -> [Urms_PCC1]
  [Iabc_PCC1] -> Bus Creator5/2  "Iabc_PCC1"
  Gain18/1 -> Sqrt10/1
  UbPCC1/1 -> Sum of Elements9/2
  Demux5/2 -> IbPCC1/1
  [Q_HVDC_to_WSCC1] -> Gain15/1
  UaPCC1/1 -> Sum of Elements9/1
  Demux5/3 -> IcPCC1/1
  Demux5/1 -> IaPCC1/1
  Sqrt10/1 -> [Irms_PCC1]
  Sum of Elements9/1 -> Gain17/1
  [Uabc_PCC1] -> Bus Creator5/1  "Uabc_PCC1"
  [P_HVDC_to_WSCC1] -> Gain14/1
  [VrmsSS1] -> VrmsSS1/1
  [PQgenSS1] -> PQgenSS1/1
  [fGenSS1] -> fGenSS1/1
  Demux1/3 -> UcPCC1/1
  IcPCC1/1 -> Sum of Elements10/3
  Demux1/1 -> UaPCC1/1
  Sum of Elements10/1 -> Gain18/1
  [PCC1_Measurements] -> PCC1_Measurements/1
  [Iabc_PCC1] -> Demux5/1
  [VabcSS1] -> VabcSS1/1
  [Uabc_PCC1] -> Demux1/1
  First-Order Filter15/1 -> Bus Creator5/3  "P_HVDC_to_WSCC1"
  First-Order Filter1/1 -> Bus Creator5/4  "Q_HVDC_to_WSCC1"
  Gain14/1 -> First-Order Filter15/1
  Gain15/1 -> First-Order Filter1/1
  First-Order Filter14/1 -> Bus Creator1/1  "V1rms"
  First-Order Filter2/1 -> Bus Creator1/2  "V2rms"
  First-Order Filter3/1 -> Bus Creator1/3  "V3rms"
  First-Order Filter4/1 -> Bus Creator1/4  "V4rms"
  First-Order Filter5/1 -> Bus Creator1/5  "V5rms"
  First-Order Filter6/1 -> Bus Creator1/6  "V6rms"
  First-Order Filter7/1 -> Bus Creator1/7  "V7rms"
  First-Order Filter8/1 -> Bus Creator1/8  "V8rms"
  First-Order Filter9/1 -> Bus Creator1/9  "V9rms"
  First-Order Filter10/1 -> Bus Creator2/1  "Pgen1"
  First-Order Filter11/1 -> Bus Creator2/2  "Qgen1"
  First-Order Filter12/1 -> Bus Creator2/3  "Pgen2"
  First-Order Filter13/1 -> Bus Creator2/4  "Qgen2"
  First-Order Filter16/1 -> Bus Creator2/5  "Pgen3"
  First-Order Filter17/1 -> Bus Creator2/6  "Qgen3"
  connections:
  Load Flow Bus6/LConn1 -- Bus_8 230 KV/RConn1 -- Line 7- 8/RConn1
  13.8 KV/230 KV 5.86 %Z/RConn1 -- Bus_9 230 KV/RConn1
  13.8 KV/230 KV 5.86 %Z/RConn2 -- Bus_9 230 KV/RConn2
  " Line 6 - 9"/RConn2 -- Bus_6 230 KV/LConn2
  Generator BUS2x1/RConn2 -- Bus_2 18 KV/LConn2
  125 MW 50 MVAR/LConn2 -- Three-Phase Breaker/RConn2 -- "Line 4 - 5 "/LConn2 -- Three-Phase V-I Measurement3/RConn2 -- Bus_5 230 KV/RConn2
  125 MW 50 MVAR/LConn3 -- Three-Phase Breaker/RConn3 -- "Line 4 - 5 "/LConn3 -- Three-Phase V-I Measurement3/RConn3 -- Bus_5 230 KV/RConn3
  "16.5 KV/230 KV 5.76 %Z     "/LConn1 -- Bus_1 16.5 KV/LConn1 -- Load Flow Bus/LConn1
  Load Flow Bus3/LConn1 -- Bus_6 230 KV/LConn1 -- " Line 6 - 9"/RConn1
  18KV/230KV 6.25 %Z/LConn1 -- Bus_2 18 KV/RConn1 -- Load Flow Bus7/LConn1
  Bus_3 13.8 KV/LConn1 -- Load Flow Bus8/LConn1 -- 13.8 KV/230 KV 5.86 %Z/LConn1
  Bus_7 230 KV/RConn6 -- Load Flow Bus4/LConn1 -- "Line 5 - 7 "/LConn1
  "16.5 KV/230 KV 5.76 %Z     "/RConn1 -- Bus_4 230 KV/LConn1 -- Load Flow Bus1/LConn1
  Bus_8 230 KV/LConn3 -- 100 MW 35 MVAR/LConn3 -- Line 8 - 9/LConn3
  "Line 5 - 7 "/RConn3 -- Bus_5 230 KV/LConn3
  125 MW 50 MVAR/LConn1 -- Three-Phase Breaker/RConn1 -- "Line 4 - 5 "/LConn1 -- Three-Phase V-I Measurement3/RConn1 -- Bus_5 230 KV/RConn1
  Generator BUS1x1/RConn1 -- Bus_1 16.5 KV/RConn1
  Bus_4 230 KV/LConn2 -- "16.5 KV/230 KV 5.76 %Z     "/RConn2
  " Line 4 - 6"/RConn2 -- Bus_4 230 KV/RConn5
  Line 7- 8/LConn2 -- Bus_7 230 KV/RConn2
  Line 8 - 9/RConn1 -- Bus_9 230 KV/LConn1
  Bus_1 16.5 KV/LConn2 -- "16.5 KV/230 KV 5.76 %Z     "/LConn2
  25 MW/LConn1 -- Three-Phase Breaker/LConn1
  18KV/230KV 6.25 %Z/RConn2 -- Bus_7 230 KV/LConn2
  Line 8 - 9/RConn2 -- Bus_9 230 KV/LConn2
  Generator BUS1x1/RConn2 -- Bus_1 16.5 KV/RConn2
  Line 7- 8/RConn3 -- Bus_8 230 KV/RConn3
  Bus_2 18 KV/RConn3 -- 18KV/230KV 6.25 %Z/LConn3
  Load Flow Bus2/LConn1 -- "Line 5 - 7 "/RConn1 -- Bus_5 230 KV/LConn1
  Bus_6 230 KV/RConn1 -- 90 MW 30 MVAR/LConn1 -- " Line 4 - 6"/LConn1
  13.8 KV/230 KV 5.86 %Z/LConn2 -- Bus_3 13.8 KV/LConn2
  Bus_6 230 KV/RConn3 -- 90 MW 30 MVAR/LConn3 -- " Line 4 - 6"/LConn3
  "16.5 KV/230 KV 5.76 %Z     "/RConn3 -- Bus_4 230 KV/LConn3
  Generator BUS1x1/RConn3 -- Bus_1 16.5 KV/RConn3
  " Line 6 - 9"/LConn1 -- Load Flow Bus5/LConn1 -- Bus_9 230 KV/LConn4
  13.8 KV/230 KV 5.86 %Z/LConn3 -- Bus_3 13.8 KV/LConn3
  Bus_6 230 KV/RConn2 -- 90 MW 30 MVAR/LConn2 -- " Line 4 - 6"/LConn2
  Line 8 - 9/RConn3 -- Bus_9 230 KV/LConn3
  Line 7- 8/RConn2 -- Bus_8 230 KV/RConn2
  18KV/230KV 6.25 %Z/LConn2 -- Bus_2 18 KV/RConn2
  13.8 KV/230 KV 5.86 %Z/RConn3 -- Bus_9 230 KV/RConn3
  Bus_8 230 KV/LConn2 -- 100 MW 35 MVAR/LConn2 -- Line 8 - 9/LConn2
  Bus_8 230 KV/LConn1 -- 100 MW 35 MVAR/LConn1 -- Line 8 - 9/LConn1
  Bus_1 16.5 KV/LConn3 -- "16.5 KV/230 KV 5.76 %Z     "/LConn3
  " Line 6 - 9"/LConn2 -- Bus_9 230 KV/LConn5
  "Line 5 - 7 "/LConn3 -- Bus_7 230 KV/RConn4
  Generator BUS3x1/RConn3 -- Bus_3 13.8 KV/RConn3
  Generator BUS3x1/RConn2 -- Bus_3 13.8 KV/RConn2
  Line 7- 8/LConn1 -- Bus_7 230 KV/RConn1
  "Line 5 - 7 "/RConn2 -- Bus_5 230 KV/LConn2
  18KV/230KV 6.25 %Z/RConn1 -- Bus_7 230 KV/LConn1
  Generator BUS3x1/RConn1 -- Bus_3 13.8 KV/RConn1
  " Line 4 - 6"/RConn1 -- Bus_4 230 KV/RConn4
  25 MW/LConn3 -- Three-Phase Breaker/LConn3
  "Line 4 - 5 "/RConn1 -- Bus_4 230 KV/RConn1
  "Line 4 - 5 "/RConn2 -- Bus_4 230 KV/RConn2
  Line 7- 8/LConn3 -- Bus_7 230 KV/RConn3
  18KV/230KV 6.25 %Z/RConn3 -- Bus_7 230 KV/LConn3
  "Line 4 - 5 "/RConn3 -- Bus_4 230 KV/RConn3
  25 MW/LConn2 -- Three-Phase Breaker/LConn2
  "Line 5 - 7 "/LConn2 -- Bus_7 230 KV/RConn5
  Generator BUS2x1/RConn3 -- Bus_2 18 KV/LConn3
  Generator BUS2x1/RConn1 -- Bus_2 18 KV/LConn1
  " Line 6 - 9"/LConn3 -- Bus_9 230 KV/LConn6
  " Line 4 - 6"/RConn3 -- Bus_4 230 KV/RConn6
  " Line 6 - 9"/RConn3 -- Bus_6 230 KV/LConn3
  Three-Phase V-I Measurement2/RConn1 -- Three-Phase V-I Measurement3/LConn1
  Three-Phase V-I Measurement2/RConn2 -- Three-Phase V-I Measurement3/LConn2
  Three-Phase V-I Measurement2/RConn3 -- Three-Phase V-I Measurement3/LConn3
  B/RConn1 -- Three-Phase V-I Measurement2/LConn2
  A/RConn1 -- Three-Phase V-I Measurement2/LConn1
  C/RConn1 -- Three-Phase V-I Measurement2/LConn3

== system HVDC_VSC_1CPUcore_dcpl/SS_HVDCStation2_WSCC2/37.5-km  cable ==
  Artemis DPL1 : Subsystem
  Artemis DPL2 : Subsystem
  BI : Subsystem  Tag=ARTEMIS model
      settings: AttributesFormatString=%<Tag>
  PM1 : PMIOPort  Port=1  Side=Left
  PM2 : PMIOPort  Port=2  Side=Right
  wires:
  Artemis DPL2/1(ho) -> Artemis DPL1/1(hi)
  Artemis DPL1/1(ho) -> Artemis DPL2/1(hi)
  connections:
  Artemis DPL2/LConn1 -- PM2/RConn1
  PM1/RConn1 -- Artemis DPL1/LConn1

== system HVDC_VSC_1CPUcore_dcpl/SS_HVDCStation2_WSCC2/37.5-km cable ==
  Artemis DPL1 : Subsystem
  Artemis DPL2 : Subsystem
  BI : Subsystem  Tag=ARTEMIS model
      settings: AttributesFormatString=%<Tag>
  PM1 : PMIOPort  Port=1  Side=Left
  PM2 : PMIOPort  Port=2  Side=Right
  wires:
  Artemis DPL1/1(ho) -> Artemis DPL2/1(hi)
  Artemis DPL2/1(ho) -> Artemis DPL1/1(hi)
  connections:
  PM1/RConn1 -- Artemis DPL1/LConn1
  Artemis DPL2/LConn1 -- PM2/RConn1

== system HVDC_VSC_1CPUcore_dcpl/SS_HVDCStation2_WSCC2/B2 ==
  Kv : Gain  Gain=Ki  SaturateOnIntegerOverflow=on  OutDataTypeStr=Inherit: Same as input  ParamDataTypeStr=Inherit: Same as input
  Kv1 : Gain  Gain=Kv  SaturateOnIntegerOverflow=on  OutDataTypeStr=Inherit: Same as input  ParamDataTypeStr=Inherit: Same as input
  Mode I : spsVIMeasurementModel/Complex
  Mode V : spsVIMeasurementModel/Complex
  Model : spsVIMeasurementModel/VI  SystemSampleTime=-1
  A : PMIOPort  Port=1  Side=Left
  B : PMIOPort  Port=2  Side=Left
  C : PMIOPort  Port=3  Side=Left
  a : PMIOPort  Port=4  Side=Right
  b : PMIOPort  Port=5  Side=Right
  c : PMIOPort  Port=6  Side=Right
  tag scope: Iabc_B2=global, Uabc_B2=global
  wires:
  Model/2 -> Kv/1
  Model/1 -> Kv1/1
  Kv/1 -> Mode I/1
  Kv1/1 -> Mode V/1
  Mode I/1 -> [Iabc_B2]
  Mode V/1 -> [Uabc_B2]
  connections:
  Model/RConn3 -- c/RConn1
  Model/RConn1 -- a/RConn1
  Model/RConn2 -- b/RConn1
  Model/LConn3 -- C/RConn1
  Model/LConn1 -- A/RConn1
  Model/LConn2 -- B/RConn1
